simulink model "RTP_15"  (R2020b)
settings: Solver=ode4  StartTime=0.0  StopTime=30  FixedStep=0.001  RelTol=1e-3
settings Model: Creator=barac  LastModifiedBy=barac

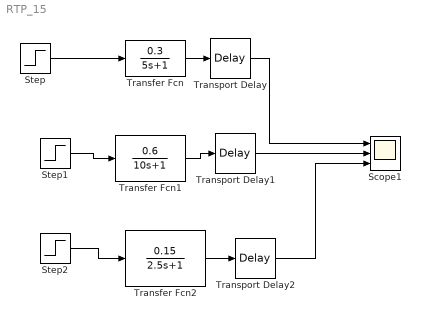
== system RTP_15 ==
  Scope1 : Scope  NumInputPorts=3
  Step : Step  After=10  SampleTime=0
  Step1 : Step  After=10  SampleTime=0
  Step2 : Step  After=10  SampleTime=0
  Transfer Fcn : TransferFcn  Numerator=[0.3]  Denominator=[5 1]
  Transfer Fcn1 : TransferFcn  Numerator=0.6  Denominator=[10 1]
  Transfer Fcn2 : TransferFcn  Numerator=[0.15]  Denominator=[2.5 1]
  Transport Delay : TransportDelay
  Transport Delay1 : TransportDelay  DelayTime=2
  Transport Delay2 : TransportDelay  DelayTime=1/2
  wires:
  Transfer Fcn/1 -> Transport Delay/1
  Step/1 -> Transfer Fcn/1
  Step1/1 -> Transfer Fcn1/1
  Transfer Fcn2/1 -> Transport Delay2/1
  Step2/1 -> Transfer Fcn2/1
  Transport Delay/1 -> Scope1/1
  Transfer Fcn1/1 -> Transport Delay1/1
  Transport Delay1/1 -> Scope1/2
  Transport Delay2/1 -> Scope1/3
